simulink model "analise_imc_planta"  (R2025a)
settings: Solver=VariableStepAuto  StartTime=0.0  StopTime=150  RelTol=1e-3
values from neighbouring files (symbols this model uses):
  Delay = 0.1    [simulink_constants.m]
  Np = 10^(-9)    (= 1e-09)    [simulink_constants.m]
  Ts = 0.5    [filtro.m]    (also in simulink_constants.m = 0.02; teste2.m)
libraries: cstblocks x3, simulink x2
settings Model: Creator=joaof  LastModifiedBy=joaof

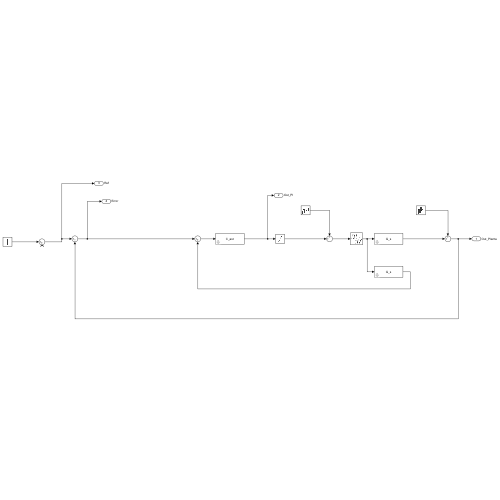
[thumbnail: Simulink's stored preview of the top-level diagram]
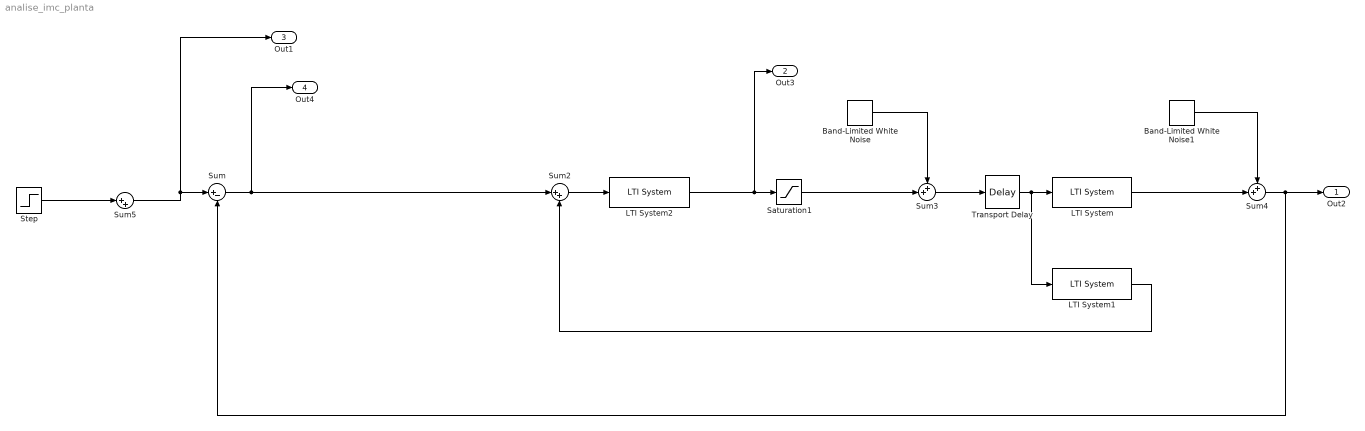
== system analise_imc_planta ==
  Band-Limited White Noise : simulink/Sources/Band-Limited White Noise  Cov=[Np]  Ts=Ts  seed=[23341]
  Band-Limited White Noise1 : simulink/Sources/Band-Limited White Noise  Cov=[Np]  Ts=Ts  seed=[23341]
  LTI System : cstblocks/LTI System  sys=G_s  IC=[]  PadeOrder=0
  LTI System1 : cstblocks/LTI System  sys=G_s  IC=[]  PadeOrder=0
  LTI System2 : cstblocks/LTI System  sys=C_ast  IC=[]  PadeOrder=0
  Saturation1 : Saturate  UpperLimit=2  LowerLimit=-2
  Step : Step  After=0.18  SampleTime=0
  Sum : Sum  Inputs=|+-
  Sum2 : Sum  Inputs=|++
  Sum3 : Sum  Inputs=++|
  Sum4 : Sum  Inputs=++|
  Sum5 : Sum  Inputs=|++
  Transport Delay : TransportDelay  DelayTime=Delay
  Out2 : Outport  SignalName=Out_Planta
  Out3 : Outport  Port=2  SignalName=Out_PI
  Out1 : Outport  Port=3  SignalName=Ref
  Out4 : Outport  Port=4  SignalName=Error
  wires:
  Band-Limited White Noise/1 -> Sum3/1
  Sum3/1 -> Transport Delay/1
  Transport Delay/1 -> LTI System1/1, LTI System/1
  LTI System/1 -> Sum4/2
  Band-Limited White Noise1/1 -> Sum4/1
  Sum4/1 -> Sum/2, Out2/1
  Sum2/1 -> LTI System2/1
  Sum/1 -> Sum2/1, Out4/1
  Step/1 -> Sum5/1
  Sum5/1 -> Out1/1, Sum/1
  Saturation1/1 -> Sum3/2
  LTI System1/1 -> Sum2/2
  LTI System2/1 -> Out3/1, Saturation1/1
